simulink model "NPC_RL_N2"  (R2017b)
settings: Solver=VariableStepAuto  StartTime=0.0  StopTime=2  MaxStep=1e-4  RelTol=1e-3
libraries: powerlib x34
settings Model: Creator=alfonso  LastModifiedBy=alfonso

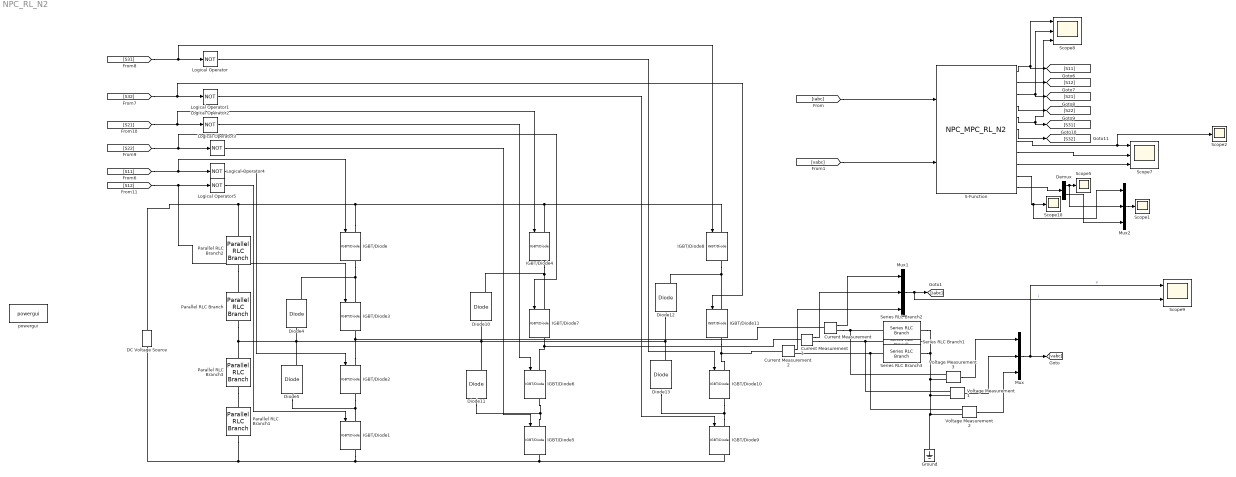
== system NPC_RL_N2 ==
  Current Measurement : powerlib/Measurements/Current Measurement  PhasorSimulation=off  OutputType=Complex  PSBequivalent=0
  Current Measurement1 : powerlib/Measurements/Current Measurement  PhasorSimulation=off  OutputType=Complex  PSBequivalent=0
  Current Measurement2 : powerlib/Measurements/Current Measurement  PhasorSimulation=off  OutputType=Complex  PSBequivalent=0
  DC Voltage Source : powerlib/Electrical Sources/DC Voltage Source  Amplitude=5200  Measurements=None
  Demux : Demux  Outputs=2
  Diode{4..5,10..13} (6 alike) : powerlib/Power Electronics/Diode  Ron=0.001  Lon=0  Vf=0.8  IC=0  UseSnubber=0  Rs=500  Cs=250e-9  Measurements=on
  Ground : powerlib/Elements/Ground  LConnTagsString=a
  IGBT/Diode{,1..11} (12 alike) : powerlib/Power Electronics/IGBT//Diode  Ron=1e-3  Rs=1e5  Cs=inf  Measurements=on
  Logical Operator{,1..5} (6 alike) : Logic  Operator=NOT  AllPortsSameDT=off  OutDataTypeStr=boolean
  Mux : Mux  Inputs=3
  Mux1 : Mux  Inputs=3
  Mux2 : Mux  Inputs=3
  Parallel RLC Branch : powerlib/Elements/Parallel RLC Branch  LConnTagsString=a  RConnTagsString=__new0  BranchType=C  Resistance=0  Inductance=0  SetiL0=off  InitialCurrent=0  Capacitance=7e-3  Setx0=off  InitialVoltage=0  Measurements=None
  Parallel RLC Branch1 : powerlib/Elements/Parallel RLC Branch  LConnTagsString=a  RConnTagsString=__new0  BranchType=C  Resistance=0  Inductance=0  SetiL0=off  InitialCurrent=0  Capacitance=7e-3  Setx0=off  InitialVoltage=0  Measurements=None
  Parallel RLC Branch2 : powerlib/Elements/Parallel RLC Branch  LConnTagsString=a  RConnTagsString=__new0  BranchType=R  Resistance=1  Inductance=0  SetiL0=off  InitialCurrent=0  Capacitance=7e-3  Setx0=off  InitialVoltage=0  Measurements=None
  Parallel RLC Branch3 : powerlib/Elements/Parallel RLC Branch  LConnTagsString=a  RConnTagsString=__new0  BranchType=R  Resistance=1  Inductance=0  SetiL0=off  InitialCurrent=0  Capacitance=7e-3  Setx0=off  InitialVoltage=0  Measurements=None
  S-Function : S-Function  FunctionName=NPC_MPC_RL_N2  SFunctionDeploymentMode=off  EnableBusSupport=off
  Scope{1..2,5,10} (4 alike) : Scope
  Scope7 : Scope  NumInputPorts=3
  Scope8 : Scope  NumInputPorts=3
  Scope9 : Scope  NumInputPorts=2
  Series RLC Branch1 : powerlib/Elements/Series RLC Branch  LConnTagsString=__new0  RConnTagsString=__new0  BranchType=RL  Resistance=2  Inductance=2e-3  SetiL0=off  InitialCurrent=0  Capacitance=0  Setx0=off  InitialVoltage=0  Measurements=None
  Series RLC Branch2 : powerlib/Elements/Series RLC Branch  LConnTagsString=__new0  RConnTagsString=__new0  BranchType=RL  Resistance=2  Inductance=2e-3  SetiL0=off  InitialCurrent=0  Capacitance=0  Setx0=off  InitialVoltage=0  Measurements=None
  Series RLC Branch3 : powerlib/Elements/Series RLC Branch  LConnTagsString=__new0  RConnTagsString=__new0  BranchType=RL  Resistance=2  Inductance=2e-3  SetiL0=off  InitialCurrent=0  Capacitance=0  Setx0=off  InitialVoltage=0  Measurements=None
  Voltage Measurement1 : powerlib/Measurements/Voltage Measurement  PhasorSimulation=off  OutputType=Complex  PSBequivalent=0
  Voltage Measurement2 : powerlib/Measurements/Voltage Measurement  PhasorSimulation=off  OutputType=Complex  PSBequivalent=0
  Voltage Measurement3 : powerlib/Measurements/Voltage Measurement  PhasorSimulation=off  OutputType=Complex  PSBequivalent=0
  powergui : powerlib/powergui  Priority=1  SimulationMode=Continuous  SampleTime=1e-6  frequency=60  Iterations=1000  frequencyindice=0  Pbase=2.035e6  ErrMax=1e-4  UnitsV=kV  UnitsW=MW  buscounter=0  FunctionMessages=off  echomessages=off  EnableUseOfTLC=off  CurrentSourceSwitches=off  DisableSnubberDevices=off  DisableRonSwitches=off  DisableVfSwitches=off  DisplayEquations=off  SolverType=Tustin/Backward Euler (TBE)  Interpol=off  ExternalGateDelay=off  methode=off  Ts=100  x0status=blocks  SPID=on  SwTol=0  HookPort=off  RestoreLinks=warning  ResistiveCurrentMeasurement=off  Frange=[0:2:500]  Ylog=off  Xlog=on  ShowGrid=off  save=off  variable=ZData  structure=corrienteN1  ZoomFFT=off  StartTime=0.05  cycles=1  DisplayStyle=1  fundamental=50  FreqAxis=off  MaxFrequency=10000  frequencyindicesteady=1  RmsSteady=1  display=off
  wires:
  Logical Operator3/1 -> IGBT/Diode5/1
  Logical Operator/1 -> IGBT/Diode10/1
  Logical Operator5/1 -> IGBT/Diode1/1
  [S21] -> Logical Operator2/1, IGBT/Diode4/1
  Logical Operator4/1 -> IGBT/Diode2/1
  [S12] -> Logical Operator5/1, IGBT/Diode3/1
  [S11] -> Logical Operator4/1, IGBT/Diode/1
  Logical Operator1/1 -> IGBT/Diode9/1
  [S22] -> Logical Operator3/1, IGBT/Diode7/1
  [S32] -> Logical Operator1/1, IGBT/Diode11/1
  Logical Operator2/1 -> IGBT/Diode6/1
  [S31] -> Logical Operator/1, IGBT/Diode8/1
  Demux/1 -> Mux2/2, Scope5/1
  S-Function/8 -> Scope7/2
  S-Function/11 -> Demux/1
  S-Function/4 -> [S22]
  S-Function/3 -> [S21], Scope8/2
  S-Function/10 -> Mux2/1, Scope10/1
  S-Function/9 -> Scope7/3
  S-Function/2 -> [S12]
  S-Function/5 -> [S31], Scope8/3
  S-Function/6 -> [S32]
  [iabc] -> S-Function/1
  S-Function/1 -> [S11], Scope8/1
  [vabc] -> S-Function/2
  Voltage Measurement3/1 -> Mux/1
  Voltage Measurement1/1 -> Mux/2
  Voltage Measurement2/1 -> Mux/3
  Mux/1 -> Scope9/1, [vabc]  "v"
  Current Measurement2/1 -> Mux1/3
  Current Measurement1/1 -> Mux1/2
  Current Measurement/1 -> Mux1/1
  Mux1/1 -> Scope9/2, [iabc]  "i"
  Demux/2 -> Mux2/3
  Mux2/1 -> Scope1/1
  S-Function/7 -> Scope2/1, Scope7/1
  connections:
  Parallel RLC Branch1/RConn1 -- DC Voltage Source/LConn1 -- IGBT/Diode5/RConn1 -- IGBT/Diode9/RConn1 -- IGBT/Diode1/RConn1
  IGBT/Diode/LConn1 -- IGBT/Diode8/LConn1 -- IGBT/Diode4/LConn1 -- Parallel RLC Branch2/LConn1 -- DC Voltage Source/RConn1
  IGBT/Diode11/RConn1 -- Current Measurement2/LConn1 -- IGBT/Diode10/LConn1
  IGBT/Diode5/LConn1 -- Diode11/LConn1 -- IGBT/Diode6/RConn1
  Diode4/RConn1 -- IGBT/Diode/RConn1 -- IGBT/Diode3/LConn1
  IGBT/Diode9/LConn1 -- Diode13/LConn1 -- IGBT/Diode10/RConn1
  IGBT/Diode4/RConn1 -- Diode10/RConn1 -- IGBT/Diode7/LConn1
  IGBT/Diode8/RConn1 -- Diode12/RConn1 -- IGBT/Diode11/LConn1
  IGBT/Diode1/LConn1 -- Diode5/LConn1 -- IGBT/Diode2/RConn1
  IGBT/Diode7/RConn1 -- Current Measurement1/LConn1 -- IGBT/Diode6/LConn1
  IGBT/Diode2/LConn1 -- Current Measurement/LConn1 -- IGBT/Diode3/RConn1
  Parallel RLC Branch3/RConn1 -- Parallel RLC Branch1/LConn1
  Parallel RLC Branch2/RConn1 -- Parallel RLC Branch/LConn1
  Current Measurement2/RConn1 -- Voltage Measurement2/LConn1 -- Series RLC Branch3/LConn1
  Current Measurement1/RConn1 -- Voltage Measurement1/LConn1 -- Series RLC Branch1/LConn1
  Current Measurement/RConn1 -- Voltage Measurement3/LConn1 -- Series RLC Branch2/LConn1
  Diode12/LConn1 -- Parallel RLC Branch3/LConn1 -- Parallel RLC Branch/RConn1 -- Diode5/RConn1 -- Diode4/LConn1 -- Diode10/LConn1 -- Diode11/RConn1 -- Diode13/RConn1
  Series RLC Branch1/RConn1 -- Voltage Measurement2/LConn2 -- Ground/LConn1 -- Voltage Measurement1/LConn2 -- Voltage Measurement3/LConn2 -- Series RLC Branch3/RConn1 -- Series RLC Branch2/RConn1
